simulink model "linearmodel"  (R2015a)
settings: Solver=ode45  StartTime=0.0  StopTime=20  FixedStep=0.01  RelTol=1e-3
values from neighbouring files (symbols this model uses):
  A = eval(As)    [Three_torque_input.m]    (also in fourinputslq_and_yaw_rate_control.m; linearization.m)
  B = eval(Bs)    [Three_torque_input.m]    (also in fourinputslq_and_yaw_rate_control.m; linearization.m)
  Kr = -inv(Cc*inv(Aa-Bb*K)*Bb)    [Three_torque_input.m]    (also in fourinputslq_and_yaw_rate_control.m = -inv(Cc*inv(Aa-Bb*K)*Bb(:,2:4)); linearization.m = -inv(sys.c*inv(sys.a-sys.b*K-eye(6))*sys.b))
undefined symbols (not defined in the file or in its folder): K, sigbuilder_block
settings Model: Creator=Jaby  LastModifiedBy=Jaby

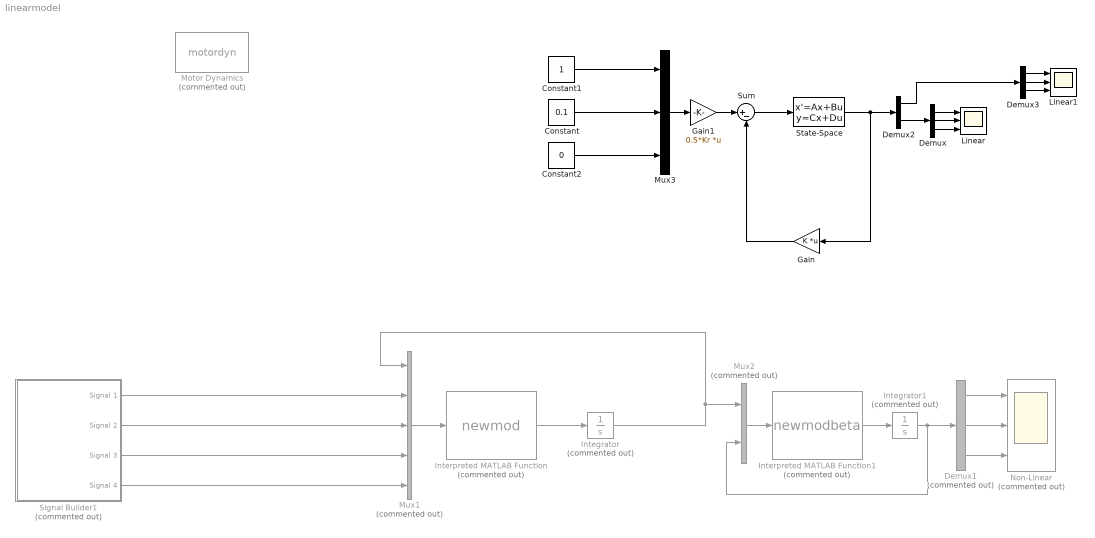
== system linearmodel ==
  Constant : Constant  Value=0.1  VectorParams1D=off
  Constant1 : Constant  VectorParams1D=off
  Constant2 : Constant  Value=0  VectorParams1D=off
  Demux : Demux  Outputs=3
  Demux1 : Demux  Commented=on  Outputs=3
  Demux2 : Demux  Outputs=2
  Demux3 : Demux  Outputs=3
  Gain : Gain  Gain=K  Multiplication=Matrix(K*u)
  Gain1 : Gain  Gain=0.5*Kr  Multiplication=Matrix(K*u)
  Integrator : Integrator  Commented=on  InitialCondition=[0 0 0]'
  Integrator1 : Integrator  Commented=on  InitialCondition=[0 0 0]'
  Interpreted MATLAB Function : MATLABFcn  Commented=on  MATLABFcn=newmod  Output1D=off
  Interpreted MATLAB Function1 : MATLABFcn  Commented=on  MATLABFcn=newmodbeta  Output1D=off
  Linear : Scope  NumInputPorts=3
      settings: TimeRange=20  YMin=0.00274~-3.07e-14~8.3e-31  YMax=0.00278~-3.025e-14~8.43e-31
  Linear1 : Scope  NumInputPorts=3
      settings: TimeRange=20  YMin=0.00274~-3.07e-14~8.3e-31  YMax=0.00278~-3.025e-14~8.43e-31  SaveName=ScopeData2
  Motor Dynamics : MATLABFcn  Commented=on  MATLABFcn=motordyn  Output1D=off
  Mux1 : Mux  Commented=on  Inputs=5
  Mux2 : Mux  Commented=on  Inputs=2
  Mux3 : Mux  Inputs=3
  "Non-Linear " : Scope  Commented=on  NumInputPorts=3
      settings: YMin=-5~-5~-5  YMax=5~5~5
  Signal Builder1 : Subsystem  Tag=STV Subsys  Commented=on  LoadFcn=sigbuilder_block('load');  StartFcn=sigbuilder_block('start');  StopFcn=sigbuilder_block('stop');  ClipboardFcn=sigbuilder_block('clipboard');  mask(Sigbuilder block){}
      mask help: Simulink:masks:SigbuilderBlock_MD
      mask init:
      | if ~strcmp(get_param(bdroot(gcbh),'SimulationStatus'),'stopped') tuvar = sigbuilder_block('maskInit'); end
      settings: CopyFcn=sigbuilder_block('copy');  DeleteFcn=sigbuilder_block('delete');  ModelCloseFcn=sigbuilder_block('modelClose');  PreSaveFcn=sigbuilder_block('preSave');  PauseFcn=sigbuilder_block('pause');  ContinueFcn=sigbuilder_block('continue');  NameChangeFcn=sigbuilder_block('namechange');  OpenFcn=sigbuilder_block('open',[437.6 199.2 550.4 400 ]);  CloseFcn=sigbuilder_block('close');
      mask Display: plot(0, 0, 100, 100,[2, 2, 32, 32, 2], [68, 8, 8, 68, 68],[32, 2], [38, 38], [32, 19, 2],[53, 60, 44], [32, 17, 17, 2],[16, 16, 31, 31]);txt = getActiveGroup(gcbh);text(2, 100, txt,'verticalAlignment', 'top');
  State-Space : StateSpace  A=A  B=B  C=eye(6)  D=zeros(6,3)  X0=0
  Sum : Sum  Inputs=|+-
  wires:
  State-Space/1 -> Demux2/1, Gain/1
  Demux/1 -> Linear/1
  Demux/2 -> Linear/2
  Demux/3 -> Linear/3
  Integrator/1 -> Mux2/1, Mux1/1
  Mux1/1 -> Interpreted MATLAB Function/1
  Interpreted MATLAB Function/1 -> Integrator/1
  Interpreted MATLAB Function1/1 -> Integrator1/1
  Demux1/2 -> "Non-Linear "/2
  Integrator1/1 -> Demux1/1, Mux2/2
  Demux1/3 -> "Non-Linear "/3
  Demux1/1 -> "Non-Linear "/1
  Mux2/1 -> Interpreted MATLAB Function1/1
  Signal Builder1/4(Signal 4) -> Mux1/5
  Signal Builder1/3(Signal 3) -> Mux1/4
  Signal Builder1/2(Signal 2) -> Mux1/3
  Signal Builder1/1(Signal 1) -> Mux1/2
  Sum/1 -> State-Space/1
  Gain/1 -> Sum/2
  Demux2/2 -> Demux/1
  Mux3/1 -> Gain1/1
  Gain1/1 -> Sum/1
  Constant/1 -> Mux3/2
  Constant1/1 -> Mux3/1
  Demux3/1 -> Linear1/1
  Demux3/2 -> Linear1/2
  Demux3/3 -> Linear1/3
  Demux2/1 -> Demux3/1
  Constant2/1 -> Mux3/3

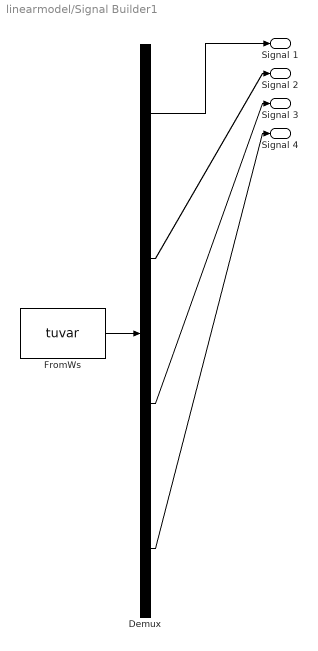
== system linearmodel/Signal Builder1 ==
  Demux : Demux  Tag=STV Demux
  FromWs : FromWorkspace  Tag=STV FromWs  VariableName=tuvar  SampleTime=0
      SigBuilderData=|
      | common.afterFinalStr = 'Extrapolate'
      | common.sampleTime = 0
      | dataSet.timeRange = [0 10]
      | dataSet.name = 'Group 1'
      | sbobj.Groups.Name = 'Group 1'
      | sbobj.Groups.Signals(1).Name = 'Signal 1'
      | sbobj.Groups.Signals(1).XData = [0 7.82 9.28 10]
      | sbobj.Groups.Signals(1).YData = [0 0 0 0]
      | sbobj.Groups.Signals(2).Name = 'Signal 2'
      | sbobj.Groups.Signals(2).XData = [0 2 2 2.1 10]
      | sbobj.Groups.Signals(2).YData = [0 0 1 1 1]
      | sbobj.Groups.Signals(3).Name = 'Signal 3'
      | sbobj.Groups.Signals(3).XData = [0 5.66 5.66 6 6 10]
      | sbobj.Groups.Signals(3).YData = [0 0 1.9 1.9 0 0]
      | sbobj.Groups.Signals(4).Name = 'Signal 4'
      | sbobj.Groups.Signals(4).XData = [0 2 2 2.1 2.1 10]
      | sbobj.Groups.Signals(4).YData = [0 0 1 1 1.35 1.35]
  Signal 1 : Outport  Tag=STV Outport
  Signal 2 : Outport  Tag=STV Outport  Port=2
  Signal 3 : Outport  Tag=STV Outport  Port=3
  Signal 4 : Outport  Tag=STV Outport  Port=4
  wires:
  Demux/1 -> Signal 1/1
  FromWs/1 -> Demux/1
  Demux/2 -> Signal 2/1
  Demux/3 -> Signal 3/1
  Demux/4 -> Signal 4/1
